simulink model "Demo_CooperativeDriving_cs"  (Simulink 7.6)
settings: Solver=ode5  SolverMode=SingleTasking  StartTime=0.0  StopTime=8  FixedStep=1/20  RelTol=1e-3
PreLoadFcn:
  | check_NUTS_defined
  | model_closed = 0;
  | assignin('base',['model_closed_' bdroot],false);
InitFcn:
  | PreScanExperimentInitFcn(bdroot)
StopFcn:
  | PreScanExperimentStopFcn(bdroot);
  | 
values from neighbouring files (symbols this model uses):
  Cf = (MLV+MRV)*g/2    (= 5460.246)    [shared_pars.m]
  Cr = (MLA+MRA)*g/2    (= 3937.734)    [shared_pars.m]
  Jzz = J_zz + 2*m_wheel*lva^2 + 2*m_wheel*laa^2    (= 3255.36268364)    [shared_pars.m]
  Kaa = 200000    [shared_pars.m]
  Kf = Kva/(g*(MLV+MRV))    (= 18.3141931701)    [shared_pars.m]
  Kr = Kaa/(g*(MLA+MRA))    (= 25.3953161895)    [shared_pars.m]
  Kva = 200000    [shared_pars.m]
  laa = l - lva    (= 1.67328601253)    [shared_pars.m]
  lva = l*(MLA+MRA)/m    (= 1.20671398747)    [shared_pars.m]
  m = MLV+MRV+MLA+MRA    (= 1916)    [shared_pars.m]
  Mu = 1    [simulinkmodel.m]
  relax_on = 0    [simulinkmodel.m]
  sigma_f = 0.65    [simulinkmodel.m]
  sigma_r = 0.65    [simulinkmodel.m]
  TyreType = 1    [simulinkmodel.m]
undefined symbols (not defined in the file or in its folder): DiscIntNeverNeededParam
libraries: PreScanSimulinkLibrary x14, PreScanUsefulBlocks x6, simulink_extras x5
(part 5 of 6)

== system Demo_CooperativeDriving_cs/Citroen_C3_1/Swarm Behavior/Vehicle Dynamics/slip_angles ==
  note: relax_on
      | ON: 1
      | OFF: 0
  dx_dy_dpsi : Inport
  delta : Inport  Port=2
  Constant : Constant  Value=relax_on
  Constant1 : Constant  Value=relax_on
  Mux2 : Mux  Inputs=2
  Sum : Sum  Inputs=++|  SaturateOnIntegerOverflow=on  InputSameDT=on  OutDataTypeStr=Inherit: Same as first input
  Switch : Switch  Threshold=0.5  SaturateOnIntegerOverflow=on  InputSameDT=on
  Switch1 : Switch  Threshold=0.5  SaturateOnIntegerOverflow=on  InputSameDT=on
  alpha_front : Fcn  Expr=-atan( (u(2)+u(3)*lva)/u(1) )
  alpha_rear : Fcn  Expr=-atan( (u(2)-u(3)*laa)/u(1) )
  relaxation_length_front : Subsystem
  relaxation_length_rear : Subsystem
  alpha : Outport
  wires:
  Constant/1 -> Switch/2
  Constant1/1 -> Switch1/2
  Switch1/1 -> Mux2/2  "alpha_r"
  Switch/1 -> Mux2/1  "alpha_f"
  relaxation_length_rear/1(alpha_relax) -> Switch1/1
  relaxation_length_front/1(alpha_relax) -> Switch/1
  alpha_rear/1 -> Switch1/3, relaxation_length_rear/1(alpha_stat)  "alpha_stat_r"
  Sum/1 -> Switch/3, relaxation_length_front/1(alpha_stat)  "alpha_stat_f"
  Mux2/1 -> alpha/1
  dx_dy_dpsi/1 -> relaxation_length_rear/2(dx,dy,dphi), alpha_rear/1, relaxation_length_front/2(dx,dy,dphi), alpha_front/1
  delta/1 -> Sum/1
  alpha_front/1 -> Sum/2

== system Demo_CooperativeDriving_cs/Citroen_C3_1/Swarm Behavior/Vehicle Dynamics/tyre_forces ==
  alpha : Inport
  delta : Inport  Port=2
  Demux1 : Demux  Outputs=2
  Fy : Fcn  Expr=u(2)*cos(u(1)) + u(3)
  M2 : Fcn  Expr=u(2)*lva*cos(u(1)) - u(3)*laa
  Mux : Mux  Inputs=2
  Mux2 : Mux  Inputs=3
  tyre_front : Subsystem
  tyre_rear : Subsystem
  Fy_wheels : Outport  InitialOutput=0
  F_lat : Outport  Port=2  InitialOutput=0
  Mz : Outport  Port=3  InitialOutput=0
  wires:
  delta/1 -> Mux2/1
  tyre_rear/1(Fy_r) -> Mux/2, Mux2/3  "Fy_r"
  tyre_front/1(Fy_f) -> Mux/1, Mux2/2  "Fy_f"
  Demux1/2 -> tyre_rear/1(alpha)
  Demux1/1 -> tyre_front/1(alpha)
  alpha/1 -> Demux1/1
  Mux2/1 -> Fy/1, M2/1
  Fy/1 -> F_lat/1
  M2/1 -> Mz/1
  Mux/1 -> Fy_wheels/1

== system Demo_CooperativeDriving_cs/Mazda_RX8_1/SELF_Demux/compas converter/cart2compas ==
  Angle [deg] : Inport
  Constant : Constant  Value=90
  Constant1 : Constant  Value=360
  Gain : Gain  Gain=1/360
  Gain1 : Gain  Gain=360
  Gain2 : Gain  Gain=-1
  Rounding Function : Rounding
  Sum : Sum  Inputs=|-+
  Sum1 : Sum  Inputs=-+|
  Sum2 : Sum  Inputs=++|
  heading [deg] : Outport
  wires:
  Sum2/1 -> heading [deg]/1
  Constant1/1 -> Sum2/1
  Gain2/1 -> Sum2/2
  Constant/1 -> Sum1/1
  Sum1/1 -> Sum/2, Gain/1
  Sum/1 -> Gain2/1
  Angle [deg]/1 -> Sum1/2
  Gain1/1 -> Sum/1
  Rounding Function/1 -> Gain1/1
  Gain/1 -> Rounding Function/1

== system Demo_CooperativeDriving_cs/Mazda_RX8_1/Trajectories/Traj2State1/Traj2State2 ==
  traj : Inport
  MuxState : Subsystem
  Traj2MuxState_Ext : Subsystem
  state : Outport
  wires:
  Traj2MuxState_Ext/9(Y [rad]) -> MuxState/9(Y [rad])
  Traj2MuxState_Ext/8(P [rad]) -> MuxState/8(P [rad])
  Traj2MuxState_Ext/7(R [rad]) -> MuxState/7(R [rad])
  Traj2MuxState_Ext/6(dz [m/s]) -> MuxState/6(dz [m/s])
  Traj2MuxState_Ext/5(dy [m/s]) -> MuxState/5(dy [m/s])
  Traj2MuxState_Ext/4(dx [m/s]) -> MuxState/4(dx [m/s])
  Traj2MuxState_Ext/3(z [m]) -> MuxState/3(z [m])
  Traj2MuxState_Ext/2(y [m]) -> MuxState/2(y [m])
  Traj2MuxState_Ext/1(x [m]) -> MuxState/1(x [m])
  MuxState/1(state) -> state/1
  traj/1 -> Traj2MuxState_Ext/1(Traj)

== system Demo_CooperativeDriving_cs/Nissan_Cabstar_1/SELF_Demux/compas converter/cart2compas ==
  Angle [deg] : Inport
  Constant : Constant  Value=90
  Constant1 : Constant  Value=360
  Gain : Gain  Gain=1/360
  Gain1 : Gain  Gain=360
  Gain2 : Gain  Gain=-1
  Rounding Function : Rounding
  Sum : Sum  Inputs=|-+
  Sum1 : Sum  Inputs=-+|
  Sum2 : Sum  Inputs=++|
  heading [deg] : Outport
  wires:
  Sum2/1 -> heading [deg]/1
  Constant1/1 -> Sum2/1
  Gain2/1 -> Sum2/2
  Constant/1 -> Sum1/1
  Sum1/1 -> Sum/2, Gain/1
  Sum/1 -> Gain2/1
  Angle [deg]/1 -> Sum1/2
  Gain1/1 -> Sum/1
  Rounding Function/1 -> Gain1/1
  Gain/1 -> Rounding Function/1

== system Demo_CooperativeDriving_cs/Nissan_Cabstar_1/Swarm Behavior/Vehicle Dynamics/eq_of_motion ==
  Vx : Inport
  F_lat : Inport  Port=2
  Mz : Inport  Port=3
  Fcn1 : Fcn  Expr=u(1)*u(3)
  Gain : Gain  Gain=1/m  SaturateOnIntegerOverflow=on  OutDataTypeStr=Inherit: Same as input  ParamDataTypeStr=Inherit: Same as input
  Gain1 : Gain  Gain=1/Jzz  SaturateOnIntegerOverflow=on  OutDataTypeStr=Inherit: Same as input  ParamDataTypeStr=Inherit: Same as input
  Integrator1 : Integrator
  Integrator4 : Integrator
  Integrator5 : Integrator
  Psip : Integrator
  Sum1 : Sum  Inputs=-+  SaturateOnIntegerOverflow=on  InputSameDT=on  OutDataTypeStr=Inherit: Same as first input
  Vx0 : Fcn  Expr=u(1)*cos(u(3)) - u(2)*sin(u(3))
  "Vy " : Integrator
  Vy0 : Fcn  Expr=u(1)*sin(u(3)) + u(2)*cos(u(3))
  X3 : Mux  Inputs=3
  Xp : Mux  Inputs=3
  Xp1 : Mux  Inputs=2
  Xp2 : Mux  Inputs=3
  x_y_psi : Outport  InitialOutput=0
  dx_dy_dpsi : Outport  Port=2  InitialOutput=0
  ddy_ddpsi : Outport  Port=3  InitialOutput=0
  wires:
  Integrator1/1 -> X3/3, Xp2/3  "psi"
  X3/1 -> x_y_psi/1
  Integrator4/1 -> X3/1  "x"
  Integrator5/1 -> X3/2  "y"
  Vy0/1 -> Integrator5/1
  Vx0/1 -> Integrator4/1
  Xp2/1 -> Vy0/1, Vx0/1
  Mz/1 -> Gain1/1
  Xp1/1 -> ddy_ddpsi/1
  F_lat/1 -> Gain/1
  Sum1/1 -> Xp1/1, "Vy "/1  "dd_y"
  Fcn1/1 -> Sum1/1
  Xp/1 -> dx_dy_dpsi/1, Fcn1/1
  Gain1/1 -> Xp1/2, Psip/1  "dd_psi"
  Vx/1 -> Xp2/1, Xp/1
  Gain/1 -> Sum1/2
  "Vy "/1 -> Xp2/2, Xp/2  "d_y"
  Psip/1 -> Integrator1/1, Xp/3  "d_psi"

== system Demo_CooperativeDriving_cs/Nissan_Cabstar_1/Swarm Behavior/Vehicle Dynamics/slip_angles ==
  note: relax_on
      | ON: 1
      | OFF: 0
  dx_dy_dpsi : Inport
  delta : Inport  Port=2
  Constant : Constant  Value=relax_on
  Constant1 : Constant  Value=relax_on
  Mux2 : Mux  Inputs=2
  Sum : Sum  Inputs=++|  SaturateOnIntegerOverflow=on  InputSameDT=on  OutDataTypeStr=Inherit: Same as first input
  Switch : Switch  Threshold=0.5  SaturateOnIntegerOverflow=on  InputSameDT=on
  Switch1 : Switch  Threshold=0.5  SaturateOnIntegerOverflow=on  InputSameDT=on
  alpha_front : Fcn  Expr=-atan( (u(2)+u(3)*lva)/u(1) )
  alpha_rear : Fcn  Expr=-atan( (u(2)-u(3)*laa)/u(1) )
  relaxation_length_front : Subsystem
  relaxation_length_rear : Subsystem
  alpha : Outport
  wires:
  Constant/1 -> Switch/2
  Constant1/1 -> Switch1/2
  Switch1/1 -> Mux2/2  "alpha_r"
  Switch/1 -> Mux2/1  "alpha_f"
  relaxation_length_rear/1(alpha_relax) -> Switch1/1
  relaxation_length_front/1(alpha_relax) -> Switch/1
  alpha_rear/1 -> Switch1/3, relaxation_length_rear/1(alpha_stat)  "alpha_stat_r"
  Sum/1 -> Switch/3, relaxation_length_front/1(alpha_stat)  "alpha_stat_f"
  Mux2/1 -> alpha/1
  dx_dy_dpsi/1 -> relaxation_length_rear/2(dx,dy,dphi), alpha_rear/1, relaxation_length_front/2(dx,dy,dphi), alpha_front/1
  delta/1 -> Sum/1
  alpha_front/1 -> Sum/2

== system Demo_CooperativeDriving_cs/Nissan_Cabstar_1/Swarm Behavior/Vehicle Dynamics/tyre_forces ==
  alpha : Inport
  delta : Inport  Port=2
  Demux1 : Demux  Outputs=2
  Fy : Fcn  Expr=u(2)*cos(u(1)) + u(3)
  M2 : Fcn  Expr=u(2)*lva*cos(u(1)) - u(3)*laa
  Mux : Mux  Inputs=2
  Mux2 : Mux  Inputs=3
  tyre_front : Subsystem
  tyre_rear : Subsystem
  Fy_wheels : Outport  InitialOutput=0
  F_lat : Outport  Port=2  InitialOutput=0
  Mz : Outport  Port=3  InitialOutput=0
  wires:
  delta/1 -> Mux2/1
  tyre_rear/1(Fy_r) -> Mux/2, Mux2/3  "Fy_r"
  tyre_front/1(Fy_f) -> Mux/1, Mux2/2  "Fy_f"
  Demux1/2 -> tyre_rear/1(alpha)
  Demux1/1 -> tyre_front/1(alpha)
  alpha/1 -> Demux1/1
  Mux2/1 -> Fy/1, M2/1
  Fy/1 -> F_lat/1
  M2/1 -> Mz/1
  Mux/1 -> Fy_wheels/1

== system Demo_CooperativeDriving_cs/Toyota_Previa_1/SELF_Demux/compas converter/cart2compas ==
  Angle [deg] : Inport
  Constant : Constant  Value=90
  Constant1 : Constant  Value=360
  Gain : Gain  Gain=1/360
  Gain1 : Gain  Gain=360
  Gain2 : Gain  Gain=-1
  Rounding Function : Rounding
  Sum : Sum  Inputs=|-+
  Sum1 : Sum  Inputs=-+|
  Sum2 : Sum  Inputs=++|
  heading [deg] : Outport
  wires:
  Sum2/1 -> heading [deg]/1
  Constant1/1 -> Sum2/1
  Gain2/1 -> Sum2/2
  Constant/1 -> Sum1/1
  Sum1/1 -> Sum/2, Gain/1
  Sum/1 -> Gain2/1
  Angle [deg]/1 -> Sum1/2
  Gain1/1 -> Sum/1
  Rounding Function/1 -> Gain1/1
  Gain/1 -> Rounding Function/1

== system Demo_CooperativeDriving_cs/Toyota_Previa_1/Swarm Behavior/Vehicle/eq_of_motion ==
  Vx : Inport
  F_lat : Inport  Port=2
  Mz : Inport  Port=3
  Fcn1 : Fcn  Expr=u(1)*u(3)
  Gain : Gain  Gain=1/m  SaturateOnIntegerOverflow=on  OutDataTypeStr=Inherit: Same as input  ParamDataTypeStr=Inherit: Same as input
  Gain1 : Gain  Gain=1/Jzz  SaturateOnIntegerOverflow=on  OutDataTypeStr=Inherit: Same as input  ParamDataTypeStr=Inherit: Same as input
  Integrator1 : Integrator
  Integrator4 : Integrator
  Integrator5 : Integrator
  Psip : Integrator
  Sum1 : Sum  Inputs=-+  SaturateOnIntegerOverflow=on  InputSameDT=on  OutDataTypeStr=Inherit: Same as first input
  Vx0 : Fcn  Expr=u(1)*cos(u(3)) - u(2)*sin(u(3))
  "Vy " : Integrator
  Vy0 : Fcn  Expr=u(1)*sin(u(3)) + u(2)*cos(u(3))
  X3 : Mux  Inputs=3
  Xp : Mux  Inputs=3
  Xp1 : Mux  Inputs=2
  Xp2 : Mux  Inputs=3
  x_y_psi : Outport  InitialOutput=0
  dx_dy_dpsi : Outport  Port=2  InitialOutput=0
  ddy_ddpsi : Outport  Port=3  InitialOutput=0
  wires:
  Integrator1/1 -> X3/3, Xp2/3  "psi"
  X3/1 -> x_y_psi/1
  Integrator4/1 -> X3/1  "x"
  Integrator5/1 -> X3/2  "y"
  Vy0/1 -> Integrator5/1
  Vx0/1 -> Integrator4/1
  Xp2/1 -> Vy0/1, Vx0/1
  Mz/1 -> Gain1/1
  Xp1/1 -> ddy_ddpsi/1
  F_lat/1 -> Gain/1
  Sum1/1 -> Xp1/1, "Vy "/1  "dd_y"
  Fcn1/1 -> Sum1/1
  Xp/1 -> dx_dy_dpsi/1, Fcn1/1
  Gain1/1 -> Xp1/2, Psip/1  "dd_psi"
  Vx/1 -> Xp2/1, Xp/1
  Gain/1 -> Sum1/2
  "Vy "/1 -> Xp2/2, Xp/2  "d_y"
  Psip/1 -> Integrator1/1, Xp/3  "d_psi"

== system Demo_CooperativeDriving_cs/Toyota_Previa_1/Swarm Behavior/Vehicle/slip_angles ==
  note: relax_on
      | ON: 1
      | OFF: 0
  dx_dy_dpsi : Inport
  delta : Inport  Port=2
  Constant : Constant  Value=relax_on
  Constant1 : Constant  Value=relax_on
  Mux2 : Mux  Inputs=2
  Sum : Sum  Inputs=++|  SaturateOnIntegerOverflow=on  InputSameDT=on  OutDataTypeStr=Inherit: Same as first input
  Switch : Switch  Threshold=0.5  SaturateOnIntegerOverflow=on  InputSameDT=on
  Switch1 : Switch  Threshold=0.5  SaturateOnIntegerOverflow=on  InputSameDT=on
  alpha_front : Fcn  Expr=-atan( (u(2)+u(3)*lva)/u(1) )
  alpha_rear : Fcn  Expr=-atan( (u(2)-u(3)*laa)/u(1) )
  relaxation_length_front : Subsystem
  relaxation_length_rear : Subsystem
  alpha : Outport
  wires:
  Constant/1 -> Switch/2
  Constant1/1 -> Switch1/2
  Switch1/1 -> Mux2/2  "alpha_r"
  Switch/1 -> Mux2/1  "alpha_f"
  relaxation_length_rear/1(alpha_relax) -> Switch1/1
  relaxation_length_front/1(alpha_relax) -> Switch/1
  alpha_rear/1 -> Switch1/3, relaxation_length_rear/1(alpha_stat)  "alpha_stat_r"
  Sum/1 -> Switch/3, relaxation_length_front/1(alpha_stat)  "alpha_stat_f"
  Mux2/1 -> alpha/1
  dx_dy_dpsi/1 -> relaxation_length_rear/2(dx,dy,dphi), alpha_rear/1, relaxation_length_front/2(dx,dy,dphi), alpha_front/1
  delta/1 -> Sum/1
  alpha_front/1 -> Sum/2

== system Demo_CooperativeDriving_cs/Toyota_Previa_1/Swarm Behavior/Vehicle/tyre_forces ==
  alpha : Inport
  delta : Inport  Port=2
  Demux1 : Demux  Outputs=2
  Fy : Fcn  Expr=u(2)*cos(u(1)) + u(3)
  M2 : Fcn  Expr=u(2)*lva*cos(u(1)) - u(3)*laa
  Mux : Mux  Inputs=2
  Mux2 : Mux  Inputs=3
  tyre_front : Subsystem
  tyre_rear : Subsystem
  Fy_wheels : Outport  InitialOutput=0
  F_lat : Outport  Port=2  InitialOutput=0
  Mz : Outport  Port=3  InitialOutput=0
  wires:
  delta/1 -> Mux2/1
  tyre_rear/1(Fy_r) -> Mux/2, Mux2/3  "Fy_r"
  tyre_front/1(Fy_f) -> Mux/1, Mux2/2  "Fy_f"
  Demux1/2 -> tyre_rear/1(alpha)
  Demux1/1 -> tyre_front/1(alpha)
  alpha/1 -> Demux1/1
  Mux2/1 -> Fy/1, M2/1
  Fy/1 -> F_lat/1
  M2/1 -> Mz/1
  Mux/1 -> Fy_wheels/1

== system Demo_CooperativeDriving_cs/Toyota_Yaris_1/SELF_Demux/compas converter/cart2compas ==
  Angle [deg] : Inport
  Constant : Constant  Value=90
  Constant1 : Constant  Value=360
  Gain : Gain  Gain=1/360
  Gain1 : Gain  Gain=360
  Gain2 : Gain  Gain=-1
  Rounding Function : Rounding
  Sum : Sum  Inputs=|-+
  Sum1 : Sum  Inputs=-+|
  Sum2 : Sum  Inputs=++|
  heading [deg] : Outport
  wires:
  Sum2/1 -> heading [deg]/1
  Constant1/1 -> Sum2/1
  Gain2/1 -> Sum2/2
  Constant/1 -> Sum1/1
  Sum1/1 -> Sum/2, Gain/1
  Sum/1 -> Gain2/1
  Angle [deg]/1 -> Sum1/2
  Gain1/1 -> Sum/1
  Rounding Function/1 -> Gain1/1
  Gain/1 -> Rounding Function/1

== system Demo_CooperativeDriving_cs/Toyota_Yaris_1/Swarm Behavior/Vehicle Dynamics/eq_of_motion ==
  Vx : Inport
  F_lat : Inport  Port=2
  Mz : Inport  Port=3
  Fcn1 : Fcn  Expr=u(1)*u(3)
  Gain : Gain  Gain=1/m  SaturateOnIntegerOverflow=on  OutDataTypeStr=Inherit: Same as input  ParamDataTypeStr=Inherit: Same as input
  Gain1 : Gain  Gain=1/Jzz  SaturateOnIntegerOverflow=on  OutDataTypeStr=Inherit: Same as input  ParamDataTypeStr=Inherit: Same as input
  Integrator1 : Integrator
  Integrator4 : Integrator
  Integrator5 : Integrator
  Psip : Integrator
  Sum1 : Sum  Inputs=-+  SaturateOnIntegerOverflow=on  InputSameDT=on  OutDataTypeStr=Inherit: Same as first input
  Vx0 : Fcn  Expr=u(1)*cos(u(3)) - u(2)*sin(u(3))
  "Vy " : Integrator
  Vy0 : Fcn  Expr=u(1)*sin(u(3)) + u(2)*cos(u(3))
  X3 : Mux  Inputs=3
  Xp : Mux  Inputs=3
  Xp1 : Mux  Inputs=2
  Xp2 : Mux  Inputs=3
  x_y_psi : Outport  InitialOutput=0
  dx_dy_dpsi : Outport  Port=2  InitialOutput=0
  ddy_ddpsi : Outport  Port=3  InitialOutput=0
  wires:
  Integrator1/1 -> X3/3, Xp2/3  "psi"
  X3/1 -> x_y_psi/1
  Integrator4/1 -> X3/1  "x"
  Integrator5/1 -> X3/2  "y"
  Vy0/1 -> Integrator5/1
  Vx0/1 -> Integrator4/1
  Xp2/1 -> Vy0/1, Vx0/1
  Mz/1 -> Gain1/1
  Xp1/1 -> ddy_ddpsi/1
  F_lat/1 -> Gain/1
  Sum1/1 -> Xp1/1, "Vy "/1  "dd_y"
  Fcn1/1 -> Sum1/1
  Xp/1 -> dx_dy_dpsi/1, Fcn1/1
  Gain1/1 -> Xp1/2, Psip/1  "dd_psi"
  Vx/1 -> Xp2/1, Xp/1
  Gain/1 -> Sum1/2
  "Vy "/1 -> Xp2/2, Xp/2  "d_y"
  Psip/1 -> Integrator1/1, Xp/3  "d_psi"

== system Demo_CooperativeDriving_cs/Toyota_Yaris_1/Swarm Behavior/Vehicle Dynamics/slip_angles ==
  note: relax_on
      | ON: 1
      | OFF: 0
  dx_dy_dpsi : Inport
  delta : Inport  Port=2
  Constant : Constant  Value=relax_on
  Constant1 : Constant  Value=relax_on
  Mux2 : Mux  Inputs=2
  Sum : Sum  Inputs=++|  SaturateOnIntegerOverflow=on  InputSameDT=on  OutDataTypeStr=Inherit: Same as first input
  Switch : Switch  Threshold=0.5  SaturateOnIntegerOverflow=on  InputSameDT=on
  Switch1 : Switch  Threshold=0.5  SaturateOnIntegerOverflow=on  InputSameDT=on
  alpha_front : Fcn  Expr=-atan( (u(2)+u(3)*lva)/u(1) )
  alpha_rear : Fcn  Expr=-atan( (u(2)-u(3)*laa)/u(1) )
  relaxation_length_front : Subsystem
  relaxation_length_rear : Subsystem
  alpha : Outport
  wires:
  Constant/1 -> Switch/2
  Constant1/1 -> Switch1/2
  Switch1/1 -> Mux2/2  "alpha_r"
  Switch/1 -> Mux2/1  "alpha_f"
  relaxation_length_rear/1(alpha_relax) -> Switch1/1
  relaxation_length_front/1(alpha_relax) -> Switch/1
  alpha_rear/1 -> Switch1/3, relaxation_length_rear/1(alpha_stat)  "alpha_stat_r"
  Sum/1 -> Switch/3, relaxation_length_front/1(alpha_stat)  "alpha_stat_f"
  Mux2/1 -> alpha/1
  dx_dy_dpsi/1 -> relaxation_length_rear/2(dx,dy,dphi), alpha_rear/1, relaxation_length_front/2(dx,dy,dphi), alpha_front/1
  delta/1 -> Sum/1
  alpha_front/1 -> Sum/2

== system Demo_CooperativeDriving_cs/Toyota_Yaris_1/Swarm Behavior/Vehicle Dynamics/tyre_forces ==
  alpha : Inport
  delta : Inport  Port=2
  Demux1 : Demux  Outputs=2
  Fy : Fcn  Expr=u(2)*cos(u(1)) + u(3)
  M2 : Fcn  Expr=u(2)*lva*cos(u(1)) - u(3)*laa
  Mux : Mux  Inputs=2
  Mux2 : Mux  Inputs=3
  tyre_front : Subsystem
  tyre_rear : Subsystem
  Fy_wheels : Outport  InitialOutput=0
  F_lat : Outport  Port=2  InitialOutput=0
  Mz : Outport  Port=3  InitialOutput=0
  wires:
  delta/1 -> Mux2/1
  tyre_rear/1(Fy_r) -> Mux/2, Mux2/3  "Fy_r"
  tyre_front/1(Fy_f) -> Mux/1, Mux2/2  "Fy_f"
  Demux1/2 -> tyre_rear/1(alpha)
  Demux1/1 -> tyre_front/1(alpha)
  alpha/1 -> Demux1/1
  Mux2/1 -> Fy/1, M2/1
  Fy/1 -> F_lat/1
  M2/1 -> Mz/1
  Mux/1 -> Fy_wheels/1

== system Demo_CooperativeDriving_cs/BMW_X5_1/Swarm Behavior/Vehicle Dynamics/slip_angles/relaxation_length_front ==
  alpha_stat : Inport
  dx,dy,dphi : Inport  Port=2
  Integrator : Integrator
  Linl : Fcn  Expr=(u(4) - u(5))/(sigma_f/u(1))
  Mux2 : Mux  Inputs={3,1,1}
  alpha_relax : Outport
  wires:
  alpha_stat/1 -> Mux2/2
  dx,dy,dphi/1 -> Mux2/1
  Integrator/1 -> Mux2/3, alpha_relax/1
  Linl/1 -> Integrator/1
  Mux2/1 -> Linl/1

== system Demo_CooperativeDriving_cs/BMW_X5_1/Swarm Behavior/Vehicle Dynamics/slip_angles/relaxation_length_rear ==
  alpha_stat : Inport
  dx,dy,dphi : Inport  Port=2
  Integrator : Integrator
  Linl : Fcn  Expr=(u(4) - u(5))/(sigma_r/u(1))
  Mux2 : Mux  Inputs={3,1,1}
  alpha_relax : Outport
  wires:
  alpha_stat/1 -> Mux2/2
  dx,dy,dphi/1 -> Mux2/1
  Integrator/1 -> Mux2/3, alpha_relax/1
  Linl/1 -> Integrator/1
  Mux2/1 -> Linl/1

== system Demo_CooperativeDriving_cs/BMW_X5_1/Swarm Behavior/Vehicle Dynamics/tyre_forces/tyre_front ==
  alpha : Inport
  Borstel : Subsystem
  Exponent : Subsystem
  Fva : Fcn  Expr=Kva*u
  Fz : Constant  Value=2*Cf
  Kf : Constant  Value=Kf
  Mu : Constant  Value=Mu
  Multiport Switch : MultiPortSwitch  zeroidx=off  SaturateOnIntegerOverflow=on  InputSameDT=on
  Type : Constant  Value=TyreType
  Fy_f : Outport  InitialOutput=0
  wires:
  Fz/1 -> Exponent/2(Fz), Borstel/2(Fz)
  Mu/1 -> Exponent/3(Mu), Borstel/3(Mu)
  alpha/1 -> Fva/1, Exponent/1(alpha), Borstel/1(alpha)
  Kf/1 -> Exponent/4(Kt), Borstel/4(Kt)
  Borstel/1(Fy) -> Multiport Switch/4
  Exponent/1(Fy) -> Multiport Switch/3
  Fva/1 -> Multiport Switch/2
  Multiport Switch/1 -> Fy_f/1
  Type/1 -> Multiport Switch/1

== system Demo_CooperativeDriving_cs/BMW_X5_1/Swarm Behavior/Vehicle Dynamics/tyre_forces/tyre_rear ==
  alpha : Inport
  Borstel : Subsystem
  Exponent : Subsystem
  Fva : Fcn  Expr=Kaa*u
  Fz : Constant  Value=2*Cr
  Kr : Constant  Value=Kr
  Mu : Constant  Value=Mu
  Multiport Switch : MultiPortSwitch  zeroidx=off  SaturateOnIntegerOverflow=on  InputSameDT=on
  Type : Constant  Value=TyreType
  Fy_r : Outport  InitialOutput=0
  wires:
  alpha/1 -> Fva/1, Exponent/1(alpha), Borstel/1(alpha)
  Fz/1 -> Exponent/2(Fz), Borstel/2(Fz)
  Mu/1 -> Exponent/3(Mu), Borstel/3(Mu)
  Kr/1 -> Exponent/4(Kt), Borstel/4(Kt)
  Borstel/1(Fy) -> Multiport Switch/4
  Exponent/1(Fy) -> Multiport Switch/3
  Fva/1 -> Multiport Switch/2
  Type/1 -> Multiport Switch/1
  Multiport Switch/1 -> Fy_r/1

== system Demo_CooperativeDriving_cs/Citroen_C3_1/Swarm Behavior/Vehicle Dynamics/slip_angles/relaxation_length_front ==
  alpha_stat : Inport
  dx,dy,dphi : Inport  Port=2
  Integrator : Integrator
  Linl : Fcn  Expr=(u(4) - u(5))/(sigma_f/u(1))
  Mux2 : Mux  Inputs={3,1,1}
  alpha_relax : Outport
  wires:
  alpha_stat/1 -> Mux2/2
  dx,dy,dphi/1 -> Mux2/1
  Integrator/1 -> Mux2/3, alpha_relax/1
  Linl/1 -> Integrator/1
  Mux2/1 -> Linl/1

== system Demo_CooperativeDriving_cs/Citroen_C3_1/Swarm Behavior/Vehicle Dynamics/slip_angles/relaxation_length_rear ==
  alpha_stat : Inport
  dx,dy,dphi : Inport  Port=2
  Integrator : Integrator
  Linl : Fcn  Expr=(u(4) - u(5))/(sigma_r/u(1))
  Mux2 : Mux  Inputs={3,1,1}
  alpha_relax : Outport
  wires:
  alpha_stat/1 -> Mux2/2
  dx,dy,dphi/1 -> Mux2/1
  Integrator/1 -> Mux2/3, alpha_relax/1
  Linl/1 -> Integrator/1
  Mux2/1 -> Linl/1

== system Demo_CooperativeDriving_cs/Citroen_C3_1/Swarm Behavior/Vehicle Dynamics/tyre_forces/tyre_front ==
  alpha : Inport
  Borstel : Subsystem
  Exponent : Subsystem
  Fva : Fcn  Expr=Kva*u
  Fz : Constant  Value=2*Cf
  Kf : Constant  Value=Kf
  Mu : Constant  Value=Mu
  Multiport Switch : MultiPortSwitch  zeroidx=off  SaturateOnIntegerOverflow=on  InputSameDT=on
  Type : Constant  Value=TyreType
  Fy_f : Outport  InitialOutput=0
  wires:
  Fz/1 -> Exponent/2(Fz), Borstel/2(Fz)
  Mu/1 -> Exponent/3(Mu), Borstel/3(Mu)
  alpha/1 -> Fva/1, Exponent/1(alpha), Borstel/1(alpha)
  Kf/1 -> Exponent/4(Kt), Borstel/4(Kt)
  Borstel/1(Fy) -> Multiport Switch/4
  Exponent/1(Fy) -> Multiport Switch/3
  Fva/1 -> Multiport Switch/2
  Multiport Switch/1 -> Fy_f/1
  Type/1 -> Multiport Switch/1

== system Demo_CooperativeDriving_cs/Citroen_C3_1/Swarm Behavior/Vehicle Dynamics/tyre_forces/tyre_rear ==
  alpha : Inport
  Borstel : Subsystem
  Exponent : Subsystem
  Fva : Fcn  Expr=Kaa*u
  Fz : Constant  Value=2*Cr
  Kr : Constant  Value=Kr
  Mu : Constant  Value=Mu
  Multiport Switch : MultiPortSwitch  zeroidx=off  SaturateOnIntegerOverflow=on  InputSameDT=on
  Type : Constant  Value=TyreType
  Fy_r : Outport  InitialOutput=0
  wires:
  alpha/1 -> Fva/1, Exponent/1(alpha), Borstel/1(alpha)
  Fz/1 -> Exponent/2(Fz), Borstel/2(Fz)
  Mu/1 -> Exponent/3(Mu), Borstel/3(Mu)
  Kr/1 -> Exponent/4(Kt), Borstel/4(Kt)
  Borstel/1(Fy) -> Multiport Switch/4
  Exponent/1(Fy) -> Multiport Switch/3
  Fva/1 -> Multiport Switch/2
  Type/1 -> Multiport Switch/1
  Multiport Switch/1 -> Fy_r/1

== system Demo_CooperativeDriving_cs/Mazda_RX8_1/Trajectories/Traj2State1/Traj2State2/MuxState ==
  x [m] : Inport
  y [m] : Inport  Port=2
  z [m] : Inport  Port=3
  dx [m/s] : Inport  Port=4
  dy [m/s] : Inport  Port=5
  dz [m/s] : Inport  Port=6
  R [rad] : Inport  Port=7
  P [rad] : Inport  Port=8
  Y [rad] : Inport  Port=9
  Mux : Mux  Inputs=9
  state : Outport
  wires:
  z [m]/1 -> Mux/3
  y [m]/1 -> Mux/2
  x [m]/1 -> Mux/1
  Y [rad]/1 -> Mux/9
  P [rad]/1 -> Mux/8
  R [rad]/1 -> Mux/7
  dz [m/s]/1 -> Mux/6
  dy [m/s]/1 -> Mux/5
  dx [m/s]/1 -> Mux/4
  Mux/1 -> state/1

== system Demo_CooperativeDriving_cs/Mazda_RX8_1/Trajectories/Traj2State1/Traj2State2/Traj2MuxState_Ext ==
  Traj : Inport
  Terminator{1..9} (9 alike) : Terminator
  demux : Subsystem
  x [m] : Outport
  y [m] : Outport  Port=2
  z [m] : Outport  Port=3
  dx [m/s] : Outport  Port=4
  dy [m/s] : Outport  Port=5
  dz [m/s] : Outport  Port=6
  R [rad] : Outport  Port=7
  P [rad] : Outport  Port=8
  Y [rad] : Outport  Port=9
  wires:
  demux/9(Y) -> Y [rad]/1
  demux/7(R) -> R [rad]/1
  demux/5(vely) -> dy [m/s]/1
  demux/4(velx) -> dx [m/s]/1
  demux/10(velR) -> Terminator4/1
  demux/11(velP) -> Terminator5/1
  demux/12(velY) -> Terminator1/1
  demux/13(accx) -> Terminator8/1
  demux/14(accy) -> Terminator9/1
  demux/15(accz) -> Terminator7/1
  demux/18(accY) -> Terminator2/1
  demux/16(accR) -> Terminator3/1
  demux/17(accP) -> Terminator6/1
  demux/3(z) -> z [m]/1
  Traj/1 -> demux/1(traj)
  demux/6(velz) -> dz [m/s]/1
  demux/1(x) -> x [m]/1
  demux/2(y) -> y [m]/1
  demux/8(P) -> P [rad]/1

== system Demo_CooperativeDriving_cs/Nissan_Cabstar_1/Swarm Behavior/Vehicle Dynamics/slip_angles/relaxation_length_front ==
  alpha_stat : Inport
  dx,dy,dphi : Inport  Port=2
  Integrator : Integrator
  Linl : Fcn  Expr=(u(4) - u(5))/(sigma_f/u(1))
  Mux2 : Mux  Inputs={3,1,1}
  alpha_relax : Outport
  wires:
  alpha_stat/1 -> Mux2/2
  dx,dy,dphi/1 -> Mux2/1
  Integrator/1 -> Mux2/3, alpha_relax/1
  Linl/1 -> Integrator/1
  Mux2/1 -> Linl/1

== system Demo_CooperativeDriving_cs/Nissan_Cabstar_1/Swarm Behavior/Vehicle Dynamics/slip_angles/relaxation_length_rear ==
  alpha_stat : Inport
  dx,dy,dphi : Inport  Port=2
  Integrator : Integrator
  Linl : Fcn  Expr=(u(4) - u(5))/(sigma_r/u(1))
  Mux2 : Mux  Inputs={3,1,1}
  alpha_relax : Outport
  wires:
  alpha_stat/1 -> Mux2/2
  dx,dy,dphi/1 -> Mux2/1
  Integrator/1 -> Mux2/3, alpha_relax/1
  Linl/1 -> Integrator/1
  Mux2/1 -> Linl/1

== system Demo_CooperativeDriving_cs/Nissan_Cabstar_1/Swarm Behavior/Vehicle Dynamics/tyre_forces/tyre_front ==
  alpha : Inport
  Borstel : Subsystem
  Exponent : Subsystem
  Fva : Fcn  Expr=Kva*u
  Fz : Constant  Value=2*Cf
  Kf : Constant  Value=Kf
  Mu : Constant  Value=Mu
  Multiport Switch : MultiPortSwitch  zeroidx=off  SaturateOnIntegerOverflow=on  InputSameDT=on
  Type : Constant  Value=TyreType
  Fy_f : Outport  InitialOutput=0
  wires:
  Fz/1 -> Exponent/2(Fz), Borstel/2(Fz)
  Mu/1 -> Exponent/3(Mu), Borstel/3(Mu)
  alpha/1 -> Fva/1, Exponent/1(alpha), Borstel/1(alpha)
  Kf/1 -> Exponent/4(Kt), Borstel/4(Kt)
  Borstel/1(Fy) -> Multiport Switch/4
  Exponent/1(Fy) -> Multiport Switch/3
  Fva/1 -> Multiport Switch/2
  Multiport Switch/1 -> Fy_f/1
  Type/1 -> Multiport Switch/1

== system Demo_CooperativeDriving_cs/Nissan_Cabstar_1/Swarm Behavior/Vehicle Dynamics/tyre_forces/tyre_rear ==
  alpha : Inport
  Borstel : Subsystem
  Exponent : Subsystem
  Fva : Fcn  Expr=Kaa*u
  Fz : Constant  Value=2*Cr
  Kr : Constant  Value=Kr
  Mu : Constant  Value=Mu
  Multiport Switch : MultiPortSwitch  zeroidx=off  SaturateOnIntegerOverflow=on  InputSameDT=on
  Type : Constant  Value=TyreType
  Fy_r : Outport  InitialOutput=0
  wires:
  alpha/1 -> Fva/1, Exponent/1(alpha), Borstel/1(alpha)
  Fz/1 -> Exponent/2(Fz), Borstel/2(Fz)
  Mu/1 -> Exponent/3(Mu), Borstel/3(Mu)
  Kr/1 -> Exponent/4(Kt), Borstel/4(Kt)
  Borstel/1(Fy) -> Multiport Switch/4
  Exponent/1(Fy) -> Multiport Switch/3
  Fva/1 -> Multiport Switch/2
  Type/1 -> Multiport Switch/1
  Multiport Switch/1 -> Fy_r/1

== system Demo_CooperativeDriving_cs/Toyota_Previa_1/Swarm Behavior/Vehicle/slip_angles/relaxation_length_front ==
  alpha_stat : Inport
  dx,dy,dphi : Inport  Port=2
  Integrator : Integrator
  Linl : Fcn  Expr=(u(4) - u(5))/(sigma_f/u(1))
  Mux2 : Mux  Inputs={3,1,1}
  alpha_relax : Outport
  wires:
  alpha_stat/1 -> Mux2/2
  dx,dy,dphi/1 -> Mux2/1
  Integrator/1 -> Mux2/3, alpha_relax/1
  Linl/1 -> Integrator/1
  Mux2/1 -> Linl/1

== system Demo_CooperativeDriving_cs/Toyota_Previa_1/Swarm Behavior/Vehicle/slip_angles/relaxation_length_rear ==
  alpha_stat : Inport
  dx,dy,dphi : Inport  Port=2
  Integrator : Integrator
  Linl : Fcn  Expr=(u(4) - u(5))/(sigma_r/u(1))
  Mux2 : Mux  Inputs={3,1,1}
  alpha_relax : Outport
  wires:
  alpha_stat/1 -> Mux2/2
  dx,dy,dphi/1 -> Mux2/1
  Integrator/1 -> Mux2/3, alpha_relax/1
  Linl/1 -> Integrator/1
  Mux2/1 -> Linl/1

== system Demo_CooperativeDriving_cs/Toyota_Previa_1/Swarm Behavior/Vehicle/tyre_forces/tyre_front ==
  alpha : Inport
  Borstel : Subsystem
  Exponent : Subsystem
  Fva : Fcn  Expr=Kva*u
  Fz : Constant  Value=2*Cf
  Kf : Constant  Value=Kf
  Mu : Constant  Value=Mu
  Multiport Switch : MultiPortSwitch  zeroidx=off  SaturateOnIntegerOverflow=on  InputSameDT=on
  Type : Constant  Value=TyreType
  Fy_f : Outport  InitialOutput=0
  wires:
  Fz/1 -> Exponent/2(Fz), Borstel/2(Fz)
  Mu/1 -> Exponent/3(Mu), Borstel/3(Mu)
  alpha/1 -> Fva/1, Exponent/1(alpha), Borstel/1(alpha)
  Kf/1 -> Exponent/4(Kt), Borstel/4(Kt)
  Borstel/1(Fy) -> Multiport Switch/4
  Exponent/1(Fy) -> Multiport Switch/3
  Fva/1 -> Multiport Switch/2
  Multiport Switch/1 -> Fy_f/1
  Type/1 -> Multiport Switch/1

== system Demo_CooperativeDriving_cs/Toyota_Previa_1/Swarm Behavior/Vehicle/tyre_forces/tyre_rear ==
  alpha : Inport
  Borstel : Subsystem
  Exponent : Subsystem
  Fva : Fcn  Expr=Kaa*u
  Fz : Constant  Value=2*Cr
  Kr : Constant  Value=Kr
  Mu : Constant  Value=Mu
  Multiport Switch : MultiPortSwitch  zeroidx=off  SaturateOnIntegerOverflow=on  InputSameDT=on
  Type : Constant  Value=TyreType
  Fy_r : Outport  InitialOutput=0
  wires:
  alpha/1 -> Fva/1, Exponent/1(alpha), Borstel/1(alpha)
  Fz/1 -> Exponent/2(Fz), Borstel/2(Fz)
  Mu/1 -> Exponent/3(Mu), Borstel/3(Mu)
  Kr/1 -> Exponent/4(Kt), Borstel/4(Kt)
  Borstel/1(Fy) -> Multiport Switch/4
  Exponent/1(Fy) -> Multiport Switch/3
  Fva/1 -> Multiport Switch/2
  Type/1 -> Multiport Switch/1
  Multiport Switch/1 -> Fy_r/1

== system Demo_CooperativeDriving_cs/Toyota_Yaris_1/Swarm Behavior/Vehicle Dynamics/slip_angles/relaxation_length_front ==
  alpha_stat : Inport
  dx,dy,dphi : Inport  Port=2
  Integrator : Integrator
  Linl : Fcn  Expr=(u(4) - u(5))/(sigma_f/u(1))
  Mux2 : Mux  Inputs={3,1,1}
  alpha_relax : Outport
  wires:
  alpha_stat/1 -> Mux2/2
  dx,dy,dphi/1 -> Mux2/1
  Integrator/1 -> Mux2/3, alpha_relax/1
  Linl/1 -> Integrator/1
  Mux2/1 -> Linl/1

== system Demo_CooperativeDriving_cs/Toyota_Yaris_1/Swarm Behavior/Vehicle Dynamics/slip_angles/relaxation_length_rear ==
  alpha_stat : Inport
  dx,dy,dphi : Inport  Port=2
  Integrator : Integrator
  Linl : Fcn  Expr=(u(4) - u(5))/(sigma_r/u(1))
  Mux2 : Mux  Inputs={3,1,1}
  alpha_relax : Outport
  wires:
  alpha_stat/1 -> Mux2/2
  dx,dy,dphi/1 -> Mux2/1
  Integrator/1 -> Mux2/3, alpha_relax/1
  Linl/1 -> Integrator/1
  Mux2/1 -> Linl/1

== system Demo_CooperativeDriving_cs/Toyota_Yaris_1/Swarm Behavior/Vehicle Dynamics/tyre_forces/tyre_front ==
  alpha : Inport
  Borstel : Subsystem
  Exponent : Subsystem
  Fva : Fcn  Expr=Kva*u
  Fz : Constant  Value=2*Cf
  Kf : Constant  Value=Kf
  Mu : Constant  Value=Mu
  Multiport Switch : MultiPortSwitch  zeroidx=off  SaturateOnIntegerOverflow=on  InputSameDT=on
  Type : Constant  Value=TyreType
  Fy_f : Outport  InitialOutput=0
  wires:
  Fz/1 -> Exponent/2(Fz), Borstel/2(Fz)
  Mu/1 -> Exponent/3(Mu), Borstel/3(Mu)
  alpha/1 -> Fva/1, Exponent/1(alpha), Borstel/1(alpha)
  Kf/1 -> Exponent/4(Kt), Borstel/4(Kt)
  Borstel/1(Fy) -> Multiport Switch/4
  Exponent/1(Fy) -> Multiport Switch/3
  Fva/1 -> Multiport Switch/2
  Multiport Switch/1 -> Fy_f/1
  Type/1 -> Multiport Switch/1

== system Demo_CooperativeDriving_cs/Toyota_Yaris_1/Swarm Behavior/Vehicle Dynamics/tyre_forces/tyre_rear ==
  alpha : Inport
  Borstel : Subsystem
  Exponent : Subsystem
  Fva : Fcn  Expr=Kaa*u
  Fz : Constant  Value=2*Cr
  Kr : Constant  Value=Kr
  Mu : Constant  Value=Mu
  Multiport Switch : MultiPortSwitch  zeroidx=off  SaturateOnIntegerOverflow=on  InputSameDT=on
  Type : Constant  Value=TyreType
  Fy_r : Outport  InitialOutput=0
  wires:
  alpha/1 -> Fva/1, Exponent/1(alpha), Borstel/1(alpha)
  Fz/1 -> Exponent/2(Fz), Borstel/2(Fz)
  Mu/1 -> Exponent/3(Mu), Borstel/3(Mu)
  Kr/1 -> Exponent/4(Kt), Borstel/4(Kt)
  Borstel/1(Fy) -> Multiport Switch/4
  Exponent/1(Fy) -> Multiport Switch/3
  Fva/1 -> Multiport Switch/2
  Type/1 -> Multiport Switch/1
  Multiport Switch/1 -> Fy_r/1

== system Demo_CooperativeDriving_cs/BMW_X5_1/Swarm Behavior/Vehicle Dynamics/tyre_forces/tyre_front/Borstel ==
  alpha : Inport
  Fz : Inport  Port=2
  Mu : Inport  Port=3
  Kt : Inport  Port=4
  Abs : Abs  SaturateOnIntegerOverflow=on
  F : Fcn  Expr=(3*u(2) - 3*u(2)^2 + u(2)^3)*u(1)
  Fmax : Fcn  Expr=u(1)
  Gain : Gain  Gain=1/3  SaturateOnIntegerOverflow=on  OutDataTypeStr=Inherit: Same as input  ParamDataTypeStr=Inherit: Same as input
  Math Function : Math  Operator=reciprocal  SaturateOnIntegerOverflow=on
  Mux1 : Mux  Inputs=2
  Product : Product  SaturateOnIntegerOverflow=on  RndMeth=Zero  InputSameDT=on  OutDataTypeStr=Inherit: Same as first input
  Product1 : Product  Inputs=3  SaturateOnIntegerOverflow=on  RndMeth=Zero  InputSameDT=on  OutDataTypeStr=Inherit: Same as first input
  Relational Operator : RelationalOperator  InputSameDT=on
  Sign : Signum
  Switch : Switch  Threshold=0.5  SaturateOnIntegerOverflow=on  InputSameDT=on
  Trigonometric Function : Trigonometry  Operator=tan
  Fy : Outport
  wires:
  Abs/1 -> Relational Operator/1, Product/1
  Kt/1 -> Gain/1
  Relational Operator/1 -> Switch/2
  Trigonometric Function/1 -> Abs/1
  Mux1/1 -> F/1, Fmax/1
  Sign/1 -> Mux1/1
  Product/1 -> Mux1/2
  F/1 -> Switch/3
  Fmax/1 -> Switch/1
  alpha/1 -> Trigonometric Function/1, Sign/1
  Switch/1 -> Product1/1
  Product1/1 -> Fy/1
  Fz/1 -> Product1/2
  Mu/1 -> Product1/3
  Gain/1 -> Product/2, Math Function/1
  Math Function/1 -> Relational Operator/2

== system Demo_CooperativeDriving_cs/BMW_X5_1/Swarm Behavior/Vehicle Dynamics/tyre_forces/tyre_front/Exponent ==
  alpha : Inport
  Fz : Inport  Port=2
  Mu : Inport  Port=3
  Kt : Inport  Port=4
  Abs : Abs  SaturateOnIntegerOverflow=on
  MuY Front Wheels : Fcn  Expr=(1 - exp(-u(2)*u(1)))
  Mux1 : Mux  Inputs=2
  Product : Product  Inputs=4  SaturateOnIntegerOverflow=on  RndMeth=Zero  InputSameDT=on  OutDataTypeStr=Inherit: Same as first input
  Saturation2 : Saturate  UpperLimit=inf  LowerLimit=1e-9
  Sign : Signum
  Fy : Outport
  wires:
  Abs/1 -> Saturation2/1
  Saturation2/1 -> Mux1/1
  Mux1/1 -> MuY Front Wheels/1
  Kt/1 -> Mux1/2
  Sign/1 -> Product/1
  MuY Front Wheels/1 -> Product/2
  alpha/1 -> Abs/1, Sign/1
  Product/1 -> Fy/1
  Fz/1 -> Product/3
  Mu/1 -> Product/4

== system Demo_CooperativeDriving_cs/BMW_X5_1/Swarm Behavior/Vehicle Dynamics/tyre_forces/tyre_rear/Borstel ==
  alpha : Inport
  Fz : Inport  Port=2
  Mu : Inport  Port=3
  Kt : Inport  Port=4
  Abs : Abs  SaturateOnIntegerOverflow=on
  F : Fcn  Expr=(3*u(2) - 3*u(2)^2 + u(2)^3)*u(1)
  Fmax : Fcn  Expr=u(1)
  Gain : Gain  Gain=1/3  SaturateOnIntegerOverflow=on  OutDataTypeStr=Inherit: Same as input  ParamDataTypeStr=Inherit: Same as input
  Math Function : Math  Operator=reciprocal  SaturateOnIntegerOverflow=on
  Mux1 : Mux  Inputs=2
  Product : Product  SaturateOnIntegerOverflow=on  RndMeth=Zero  InputSameDT=on  OutDataTypeStr=Inherit: Same as first input
  Product1 : Product  Inputs=3  SaturateOnIntegerOverflow=on  RndMeth=Zero  InputSameDT=on  OutDataTypeStr=Inherit: Same as first input
  Relational Operator : RelationalOperator  InputSameDT=on
  Sign : Signum
  Switch : Switch  Threshold=0.5  SaturateOnIntegerOverflow=on  InputSameDT=on
  Trigonometric Function : Trigonometry  Operator=tan
  Fy : Outport
  wires:
  Abs/1 -> Relational Operator/1, Product/1
  Kt/1 -> Gain/1
  Relational Operator/1 -> Switch/2
  Trigonometric Function/1 -> Abs/1
  Mux1/1 -> F/1, Fmax/1
  Sign/1 -> Mux1/1
  Product/1 -> Mux1/2
  F/1 -> Switch/3
  Fmax/1 -> Switch/1
  alpha/1 -> Trigonometric Function/1, Sign/1
  Switch/1 -> Product1/1
  Product1/1 -> Fy/1
  Fz/1 -> Product1/2
  Mu/1 -> Product1/3
  Gain/1 -> Product/2, Math Function/1
  Math Function/1 -> Relational Operator/2

== system Demo_CooperativeDriving_cs/BMW_X5_1/Swarm Behavior/Vehicle Dynamics/tyre_forces/tyre_rear/Exponent ==
  alpha : Inport
  Fz : Inport  Port=2
  Mu : Inport  Port=3
  Kt : Inport  Port=4
  Abs : Abs  SaturateOnIntegerOverflow=on
  MuY Front Wheels : Fcn  Expr=(1 - exp(-u(2)*u(1)))
  Mux1 : Mux  Inputs=2
  Product : Product  Inputs=4  SaturateOnIntegerOverflow=on  RndMeth=Zero  InputSameDT=on  OutDataTypeStr=Inherit: Same as first input
  Saturation2 : Saturate  UpperLimit=inf  LowerLimit=1e-9
  Sign : Signum
  Fy : Outport
  wires:
  Abs/1 -> Saturation2/1
  Saturation2/1 -> Mux1/1
  Mux1/1 -> MuY Front Wheels/1
  Kt/1 -> Mux1/2
  Sign/1 -> Product/1
  MuY Front Wheels/1 -> Product/2
  alpha/1 -> Abs/1, Sign/1
  Product/1 -> Fy/1
  Fz/1 -> Product/3
  Mu/1 -> Product/4

== system Demo_CooperativeDriving_cs/Citroen_C3_1/Swarm Behavior/Vehicle Dynamics/tyre_forces/tyre_front/Borstel ==
  alpha : Inport
  Fz : Inport  Port=2
  Mu : Inport  Port=3
  Kt : Inport  Port=4
  Abs : Abs  SaturateOnIntegerOverflow=on
  F : Fcn  Expr=(3*u(2) - 3*u(2)^2 + u(2)^3)*u(1)
  Fmax : Fcn  Expr=u(1)
  Gain : Gain  Gain=1/3  SaturateOnIntegerOverflow=on  OutDataTypeStr=Inherit: Same as input  ParamDataTypeStr=Inherit: Same as input
  Math Function : Math  Operator=reciprocal  SaturateOnIntegerOverflow=on
  Mux1 : Mux  Inputs=2
  Product : Product  SaturateOnIntegerOverflow=on  RndMeth=Zero  InputSameDT=on  OutDataTypeStr=Inherit: Same as first input
  Product1 : Product  Inputs=3  SaturateOnIntegerOverflow=on  RndMeth=Zero  InputSameDT=on  OutDataTypeStr=Inherit: Same as first input
  Relational Operator : RelationalOperator  InputSameDT=on
  Sign : Signum
  Switch : Switch  Threshold=0.5  SaturateOnIntegerOverflow=on  InputSameDT=on
  Trigonometric Function : Trigonometry  Operator=tan
  Fy : Outport
  wires:
  Abs/1 -> Relational Operator/1, Product/1
  Kt/1 -> Gain/1
  Relational Operator/1 -> Switch/2
  Trigonometric Function/1 -> Abs/1
  Mux1/1 -> F/1, Fmax/1
  Sign/1 -> Mux1/1
  Product/1 -> Mux1/2
  F/1 -> Switch/3
  Fmax/1 -> Switch/1
  alpha/1 -> Trigonometric Function/1, Sign/1
  Switch/1 -> Product1/1
  Product1/1 -> Fy/1
  Fz/1 -> Product1/2
  Mu/1 -> Product1/3
  Gain/1 -> Product/2, Math Function/1
  Math Function/1 -> Relational Operator/2

== system Demo_CooperativeDriving_cs/Citroen_C3_1/Swarm Behavior/Vehicle Dynamics/tyre_forces/tyre_front/Exponent ==
  alpha : Inport
  Fz : Inport  Port=2
  Mu : Inport  Port=3
  Kt : Inport  Port=4
  Abs : Abs  SaturateOnIntegerOverflow=on
  MuY Front Wheels : Fcn  Expr=(1 - exp(-u(2)*u(1)))
  Mux1 : Mux  Inputs=2
  Product : Product  Inputs=4  SaturateOnIntegerOverflow=on  RndMeth=Zero  InputSameDT=on  OutDataTypeStr=Inherit: Same as first input
  Saturation2 : Saturate  UpperLimit=inf  LowerLimit=1e-9
  Sign : Signum
  Fy : Outport
  wires:
  Abs/1 -> Saturation2/1
  Saturation2/1 -> Mux1/1
  Mux1/1 -> MuY Front Wheels/1
  Kt/1 -> Mux1/2
  Sign/1 -> Product/1
  MuY Front Wheels/1 -> Product/2
  alpha/1 -> Abs/1, Sign/1
  Product/1 -> Fy/1
  Fz/1 -> Product/3
  Mu/1 -> Product/4

== system Demo_CooperativeDriving_cs/Citroen_C3_1/Swarm Behavior/Vehicle Dynamics/tyre_forces/tyre_rear/Borstel ==
  alpha : Inport
  Fz : Inport  Port=2
  Mu : Inport  Port=3
  Kt : Inport  Port=4
  Abs : Abs  SaturateOnIntegerOverflow=on
  F : Fcn  Expr=(3*u(2) - 3*u(2)^2 + u(2)^3)*u(1)
  Fmax : Fcn  Expr=u(1)
  Gain : Gain  Gain=1/3  SaturateOnIntegerOverflow=on  OutDataTypeStr=Inherit: Same as input  ParamDataTypeStr=Inherit: Same as input
  Math Function : Math  Operator=reciprocal  SaturateOnIntegerOverflow=on
  Mux1 : Mux  Inputs=2
  Product : Product  SaturateOnIntegerOverflow=on  RndMeth=Zero  InputSameDT=on  OutDataTypeStr=Inherit: Same as first input
  Product1 : Product  Inputs=3  SaturateOnIntegerOverflow=on  RndMeth=Zero  InputSameDT=on  OutDataTypeStr=Inherit: Same as first input
  Relational Operator : RelationalOperator  InputSameDT=on
  Sign : Signum
  Switch : Switch  Threshold=0.5  SaturateOnIntegerOverflow=on  InputSameDT=on
  Trigonometric Function : Trigonometry  Operator=tan
  Fy : Outport
  wires:
  Abs/1 -> Relational Operator/1, Product/1
  Kt/1 -> Gain/1
  Relational Operator/1 -> Switch/2
  Trigonometric Function/1 -> Abs/1
  Mux1/1 -> F/1, Fmax/1
  Sign/1 -> Mux1/1
  Product/1 -> Mux1/2
  F/1 -> Switch/3
  Fmax/1 -> Switch/1
  alpha/1 -> Trigonometric Function/1, Sign/1
  Switch/1 -> Product1/1
  Product1/1 -> Fy/1
  Fz/1 -> Product1/2
  Mu/1 -> Product1/3
  Gain/1 -> Product/2, Math Function/1
  Math Function/1 -> Relational Operator/2

== system Demo_CooperativeDriving_cs/Citroen_C3_1/Swarm Behavior/Vehicle Dynamics/tyre_forces/tyre_rear/Exponent ==
  alpha : Inport
  Fz : Inport  Port=2
  Mu : Inport  Port=3
  Kt : Inport  Port=4
  Abs : Abs  SaturateOnIntegerOverflow=on
  MuY Front Wheels : Fcn  Expr=(1 - exp(-u(2)*u(1)))
  Mux1 : Mux  Inputs=2
  Product : Product  Inputs=4  SaturateOnIntegerOverflow=on  RndMeth=Zero  InputSameDT=on  OutDataTypeStr=Inherit: Same as first input
  Saturation2 : Saturate  UpperLimit=inf  LowerLimit=1e-9
  Sign : Signum
  Fy : Outport
  wires:
  Abs/1 -> Saturation2/1
  Saturation2/1 -> Mux1/1
  Mux1/1 -> MuY Front Wheels/1
  Kt/1 -> Mux1/2
  Sign/1 -> Product/1
  MuY Front Wheels/1 -> Product/2
  alpha/1 -> Abs/1, Sign/1
  Product/1 -> Fy/1
  Fz/1 -> Product/3
  Mu/1 -> Product/4

== system Demo_CooperativeDriving_cs/Mazda_RX8_1/Trajectories/Traj2State1/Traj2State2/Traj2MuxState_Ext/demux ==
  traj : Inport
  Demux : Demux  Outputs=18
  x : Outport
  y : Outport  Port=2
  z : Outport  Port=3
  velx : Outport  Port=4
  vely : Outport  Port=5
  velz : Outport  Port=6
  R : Outport  Port=7
  P : Outport  Port=8
  Y : Outport  Port=9
  velR : Outport  Port=10
  velP : Outport  Port=11
  velY : Outport  Port=12
  accx : Outport  Port=13
  accy : Outport  Port=14
  accz : Outport  Port=15
  accR : Outport  Port=16
  accP : Outport  Port=17
  accY : Outport  Port=18
  wires:
  Demux/18 -> accY/1
  Demux/17 -> accP/1
  Demux/16 -> accR/1
  Demux/15 -> accz/1
  Demux/14 -> accy/1
  Demux/13 -> accx/1
  Demux/12 -> velY/1
  Demux/11 -> velP/1
  Demux/10 -> velR/1
  Demux/9 -> velz/1
  Demux/8 -> vely/1
  Demux/7 -> velx/1
  Demux/6 -> Y/1
  Demux/5 -> P/1
  traj/1 -> Demux/1
  Demux/4 -> R/1
  Demux/3 -> z/1
  Demux/2 -> y/1
  Demux/1 -> x/1

== system Demo_CooperativeDriving_cs/Nissan_Cabstar_1/Swarm Behavior/Vehicle Dynamics/tyre_forces/tyre_front/Borstel ==
  alpha : Inport
  Fz : Inport  Port=2
  Mu : Inport  Port=3
  Kt : Inport  Port=4
  Abs : Abs  SaturateOnIntegerOverflow=on
  F : Fcn  Expr=(3*u(2) - 3*u(2)^2 + u(2)^3)*u(1)
  Fmax : Fcn  Expr=u(1)
  Gain : Gain  Gain=1/3  SaturateOnIntegerOverflow=on  OutDataTypeStr=Inherit: Same as input  ParamDataTypeStr=Inherit: Same as input
  Math Function : Math  Operator=reciprocal  SaturateOnIntegerOverflow=on
  Mux1 : Mux  Inputs=2
  Product : Product  SaturateOnIntegerOverflow=on  RndMeth=Zero  InputSameDT=on  OutDataTypeStr=Inherit: Same as first input
  Product1 : Product  Inputs=3  SaturateOnIntegerOverflow=on  RndMeth=Zero  InputSameDT=on  OutDataTypeStr=Inherit: Same as first input
  Relational Operator : RelationalOperator  InputSameDT=on
  Sign : Signum
  Switch : Switch  Threshold=0.5  SaturateOnIntegerOverflow=on  InputSameDT=on
  Trigonometric Function : Trigonometry  Operator=tan
  Fy : Outport
  wires:
  Abs/1 -> Relational Operator/1, Product/1
  Kt/1 -> Gain/1
  Relational Operator/1 -> Switch/2
  Trigonometric Function/1 -> Abs/1
  Mux1/1 -> F/1, Fmax/1
  Sign/1 -> Mux1/1
  Product/1 -> Mux1/2
  F/1 -> Switch/3
  Fmax/1 -> Switch/1
  alpha/1 -> Trigonometric Function/1, Sign/1
  Switch/1 -> Product1/1
  Product1/1 -> Fy/1
  Fz/1 -> Product1/2
  Mu/1 -> Product1/3
  Gain/1 -> Product/2, Math Function/1
  Math Function/1 -> Relational Operator/2

== system Demo_CooperativeDriving_cs/Nissan_Cabstar_1/Swarm Behavior/Vehicle Dynamics/tyre_forces/tyre_front/Exponent ==
  alpha : Inport
  Fz : Inport  Port=2
  Mu : Inport  Port=3
  Kt : Inport  Port=4
  Abs : Abs  SaturateOnIntegerOverflow=on
  MuY Front Wheels : Fcn  Expr=(1 - exp(-u(2)*u(1)))
  Mux1 : Mux  Inputs=2
  Product : Product  Inputs=4  SaturateOnIntegerOverflow=on  RndMeth=Zero  InputSameDT=on  OutDataTypeStr=Inherit: Same as first input
  Saturation2 : Saturate  UpperLimit=inf  LowerLimit=1e-9
  Sign : Signum
  Fy : Outport
  wires:
  Abs/1 -> Saturation2/1
  Saturation2/1 -> Mux1/1
  Mux1/1 -> MuY Front Wheels/1
  Kt/1 -> Mux1/2
  Sign/1 -> Product/1
  MuY Front Wheels/1 -> Product/2
  alpha/1 -> Abs/1, Sign/1
  Product/1 -> Fy/1
  Fz/1 -> Product/3
  Mu/1 -> Product/4

== system Demo_CooperativeDriving_cs/Nissan_Cabstar_1/Swarm Behavior/Vehicle Dynamics/tyre_forces/tyre_rear/Borstel ==
  alpha : Inport
  Fz : Inport  Port=2
  Mu : Inport  Port=3
  Kt : Inport  Port=4
  Abs : Abs  SaturateOnIntegerOverflow=on
  F : Fcn  Expr=(3*u(2) - 3*u(2)^2 + u(2)^3)*u(1)
  Fmax : Fcn  Expr=u(1)
  Gain : Gain  Gain=1/3  SaturateOnIntegerOverflow=on  OutDataTypeStr=Inherit: Same as input  ParamDataTypeStr=Inherit: Same as input
  Math Function : Math  Operator=reciprocal  SaturateOnIntegerOverflow=on
  Mux1 : Mux  Inputs=2
  Product : Product  SaturateOnIntegerOverflow=on  RndMeth=Zero  InputSameDT=on  OutDataTypeStr=Inherit: Same as first input
  Product1 : Product  Inputs=3  SaturateOnIntegerOverflow=on  RndMeth=Zero  InputSameDT=on  OutDataTypeStr=Inherit: Same as first input
  Relational Operator : RelationalOperator  InputSameDT=on
  Sign : Signum
  Switch : Switch  Threshold=0.5  SaturateOnIntegerOverflow=on  InputSameDT=on
  Trigonometric Function : Trigonometry  Operator=tan
  Fy : Outport
  wires:
  Abs/1 -> Relational Operator/1, Product/1
  Kt/1 -> Gain/1
  Relational Operator/1 -> Switch/2
  Trigonometric Function/1 -> Abs/1
  Mux1/1 -> F/1, Fmax/1
  Sign/1 -> Mux1/1
  Product/1 -> Mux1/2
  F/1 -> Switch/3
  Fmax/1 -> Switch/1
  alpha/1 -> Trigonometric Function/1, Sign/1
  Switch/1 -> Product1/1
  Product1/1 -> Fy/1
  Fz/1 -> Product1/2
  Mu/1 -> Product1/3
  Gain/1 -> Product/2, Math Function/1
  Math Function/1 -> Relational Operator/2

== system Demo_CooperativeDriving_cs/Nissan_Cabstar_1/Swarm Behavior/Vehicle Dynamics/tyre_forces/tyre_rear/Exponent ==
  alpha : Inport
  Fz : Inport  Port=2
  Mu : Inport  Port=3
  Kt : Inport  Port=4
  Abs : Abs  SaturateOnIntegerOverflow=on
  MuY Front Wheels : Fcn  Expr=(1 - exp(-u(2)*u(1)))
  Mux1 : Mux  Inputs=2
  Product : Product  Inputs=4  SaturateOnIntegerOverflow=on  RndMeth=Zero  InputSameDT=on  OutDataTypeStr=Inherit: Same as first input
  Saturation2 : Saturate  UpperLimit=inf  LowerLimit=1e-9
  Sign : Signum
  Fy : Outport
  wires:
  Abs/1 -> Saturation2/1
  Saturation2/1 -> Mux1/1
  Mux1/1 -> MuY Front Wheels/1
  Kt/1 -> Mux1/2
  Sign/1 -> Product/1
  MuY Front Wheels/1 -> Product/2
  alpha/1 -> Abs/1, Sign/1
  Product/1 -> Fy/1
  Fz/1 -> Product/3
  Mu/1 -> Product/4

== system Demo_CooperativeDriving_cs/Toyota_Previa_1/Swarm Behavior/Vehicle/tyre_forces/tyre_front/Borstel ==
  alpha : Inport
  Fz : Inport  Port=2
  Mu : Inport  Port=3
  Kt : Inport  Port=4
  Abs : Abs  SaturateOnIntegerOverflow=on
  F : Fcn  Expr=(3*u(2) - 3*u(2)^2 + u(2)^3)*u(1)
  Fmax : Fcn  Expr=u(1)
  Gain : Gain  Gain=1/3  SaturateOnIntegerOverflow=on  OutDataTypeStr=Inherit: Same as input  ParamDataTypeStr=Inherit: Same as input
  Math Function : Math  Operator=reciprocal  SaturateOnIntegerOverflow=on
  Mux1 : Mux  Inputs=2
  Product : Product  SaturateOnIntegerOverflow=on  RndMeth=Zero  InputSameDT=on  OutDataTypeStr=Inherit: Same as first input
  Product1 : Product  Inputs=3  SaturateOnIntegerOverflow=on  RndMeth=Zero  InputSameDT=on  OutDataTypeStr=Inherit: Same as first input
  Relational Operator : RelationalOperator  InputSameDT=on
  Sign : Signum
  Switch : Switch  Threshold=0.5  SaturateOnIntegerOverflow=on  InputSameDT=on
  Trigonometric Function : Trigonometry  Operator=tan
  Fy : Outport
  wires:
  Abs/1 -> Relational Operator/1, Product/1
  Kt/1 -> Gain/1
  Relational Operator/1 -> Switch/2
  Trigonometric Function/1 -> Abs/1
  Mux1/1 -> F/1, Fmax/1
  Sign/1 -> Mux1/1
  Product/1 -> Mux1/2
  F/1 -> Switch/3
  Fmax/1 -> Switch/1
  alpha/1 -> Trigonometric Function/1, Sign/1
  Switch/1 -> Product1/1
  Product1/1 -> Fy/1
  Fz/1 -> Product1/2
  Mu/1 -> Product1/3
  Gain/1 -> Product/2, Math Function/1
  Math Function/1 -> Relational Operator/2

== system Demo_CooperativeDriving_cs/Toyota_Previa_1/Swarm Behavior/Vehicle/tyre_forces/tyre_front/Exponent ==
  alpha : Inport
  Fz : Inport  Port=2
  Mu : Inport  Port=3
  Kt : Inport  Port=4
  Abs : Abs  SaturateOnIntegerOverflow=on
  MuY Front Wheels : Fcn  Expr=(1 - exp(-u(2)*u(1)))
  Mux1 : Mux  Inputs=2
  Product : Product  Inputs=4  SaturateOnIntegerOverflow=on  RndMeth=Zero  InputSameDT=on  OutDataTypeStr=Inherit: Same as first input
  Saturation2 : Saturate  UpperLimit=inf  LowerLimit=1e-9
  Sign : Signum
  Fy : Outport
  wires:
  Abs/1 -> Saturation2/1
  Saturation2/1 -> Mux1/1
  Mux1/1 -> MuY Front Wheels/1
  Kt/1 -> Mux1/2
  Sign/1 -> Product/1
  MuY Front Wheels/1 -> Product/2
  alpha/1 -> Abs/1, Sign/1
  Product/1 -> Fy/1
  Fz/1 -> Product/3
  Mu/1 -> Product/4
